simulink model "Askhsh_12b"  (R2018b)
settings: Solver=VariableStepAuto  StartTime=0.0  StopTime=10  RelTol=1e-3
settings Model: Creator=Argy  LastModifiedBy=Argy
settings DataIOCC: Refine=10

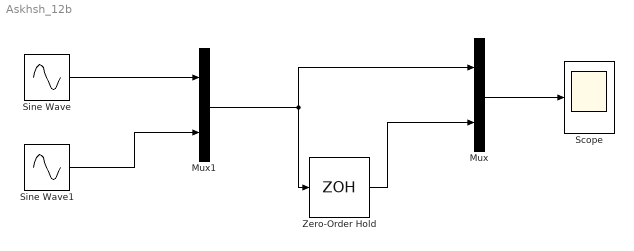
== system Askhsh_12b ==
  Mux : Mux  Inputs=2
  Mux1 : Mux  Inputs=2
  Scope : Scope
  Sine Wave : Sin  Amplitude=4  Frequency=10  SampleTime=0
  Sine Wave1 : Sin  Amplitude=2  Frequency=5  SampleTime=0
  Zero-Order Hold : ZeroOrderHold  SampleTime=0.2
  wires:
  Mux/1 -> Scope/1
  Zero-Order Hold/1 -> Mux/2
  Sine Wave/1 -> Mux1/1
  Sine Wave1/1 -> Mux1/2
  Mux1/1 -> Zero-Order Hold/1, Mux/1
